simulink model "sensorfusion_diffdrive_VW"  (R2020b)
settings: Solver=ode1  StartTime=0.0  StopTime=100  FixedStep=0.01  RelTol=1e-3
settings Model: Creator=ONLY-GOD  LastModifiedBy=ONLY-GOD

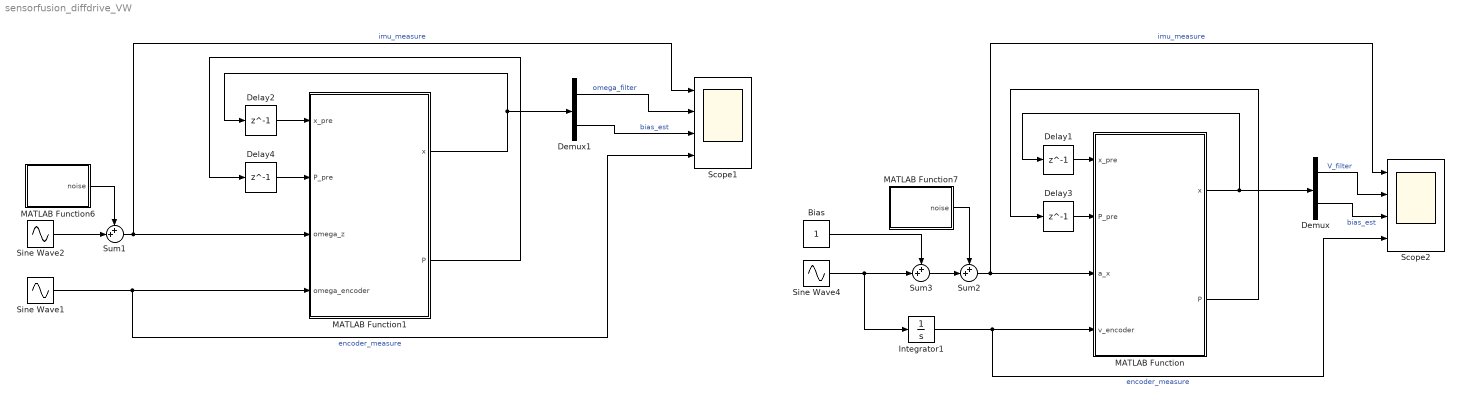
== system sensorfusion_diffdrive_VW ==
  Bias : Constant
  Delay1 : Delay  DelayLength=1  InitialCondition=[0;0]
  Delay2 : Delay  DelayLength=1  InitialCondition=[0;0]
  Delay3 : Delay  DelayLength=1  InitialCondition=2*eye(2);
  Delay4 : Delay  DelayLength=1  InitialCondition=2*eye(2);
  Demux : Demux  Outputs=2
  Demux1 : Demux  Outputs=2
  Integrator1 : Integrator
  MATLAB Function : MATLAB Function  TreatAsAtomicUnit=on
  MATLAB Function1 : MATLAB Function  TreatAsAtomicUnit=on
  MATLAB Function6 : MATLAB Function  TreatAsAtomicUnit=on
  MATLAB Function7 : MATLAB Function  TreatAsAtomicUnit=on
  Scope1 : Scope  NumInputPorts=4
  Scope2 : Scope  NumInputPorts=4
  Sine Wave1 : Sin  Amplitude=5  Frequency=0.1
  Sine Wave2 : Sin  Amplitude=5  Bias=1  Frequency=0.1
  Sine Wave4 : Sin  Amplitude=5  Frequency=0.1
  Sum1 : Sum  Inputs=++|
  Sum2 : Sum  Inputs=++|
  Sum3 : Sum  Inputs=++|
  wires:
  MATLAB Function/1(x) -> Delay1/1, Demux/1
  Demux/1 -> Scope2/2  "V_filter"
  Demux/2 -> Scope2/3  "bias_est"
  MATLAB Function/2(P) -> Delay3/1
  Delay3/1 -> MATLAB Function/2(P_pre)
  Delay1/1 -> MATLAB Function/1(x_pre)
  Delay2/1 -> MATLAB Function1/1(x_pre)
  MATLAB Function1/2(P) -> Delay4/1
  MATLAB Function1/1(x) -> Demux1/1, Delay2/1
  Delay4/1 -> MATLAB Function1/2(P_pre)
  Demux1/2 -> Scope1/3  "bias_est"
  Sine Wave1/1 -> Scope1/4, MATLAB Function1/4(omega_encoder)  "encoder_measure"
  Sum1/1 -> Scope1/1, MATLAB Function1/3(omega_z)  "imu_measure"
  Demux1/1 -> Scope1/2  "omega_filter"
  Sum2/1 -> Scope2/1, MATLAB Function/3(a_x)  "imu_measure"
  Integrator1/1 -> Scope2/4, MATLAB Function/4(v_encoder)  "encoder_measure"
  MATLAB Function7/1(noise) -> Sum2/1
  Sum3/1 -> Sum2/2
  Sine Wave4/1 -> Sum3/2, Integrator1/1
  Bias/1 -> Sum3/1
  Sine Wave2/1 -> Sum1/2
  MATLAB Function6/1(noise) -> Sum1/1

== matlab function sensorfusion_diffdrive_VW/MATLAB Function ==
  data: x_pre input; P_pre input; a_x input; x output; v_encoder input; P output
function [x,P] = kalman_V(x_pre,P_pre,a_x,v_encoder)
% predefined
Ts = 0.01;
Q = 1e-1*diag([2 2]);
R = 1e-3;
% model prediction
A = [1 Ts;
     0 1];
B = [Ts;
     0];
C = [1 0];

u = a_x;

x = A*x_pre + B*u;   %(2x1) = (2x2)(2x1) + (2x1)(1x1) checked
P = A*P_pre*A' + Q;  %(2x2) = (2x2)(2x2)(2x2) + (2x2) checked

%update
erry = v_encoder - C*x;      %(1x1) = (1x1) + (1x2)(2x1) checked
P_xz = P*C';
P_zz = C*P*C' + R;
x = x + (P_xz/P_zz)*erry;
P = P - (P_xz/P_zz)*P_xz';

== matlab function sensorfusion_diffdrive_VW/MATLAB Function1 ==
  data: x_pre input; P_pre input; omega_z input; x output; omega_encoder input; P output
function [x,P] = kalman_omega(x_pre,P_pre,omega_z,omega_encoder)
% predefined
Ts = 0.01;
Q = 1e-1*diag([2 200]);
R = 1e-4;
% model prediction
A = [0 1;
     0 1];
B = [1;
     0];
C = [1 0];

u = omega_z;

x = A*x_pre + B*u;   %(2x1) = (2x2)(2x1) + (2x1)(1x1) checked
P = A*P_pre*A' + Q;  %(2x2) = (2x2)(2x2)(2x2) + (2x2) checked

%update
erry = omega_encoder - C*x;      %(1x1) = (1x1) + (1x2)(2x1) checked
P_xz = P*C';
P_zz = C*P*C' + R;
x = x + (P_xz/P_zz)*erry;
P = P - (P_xz/P_zz)*P_xz';

== matlab function sensorfusion_diffdrive_VW/MATLAB Function6 ==
  data: noise output
function noise = fnc()

noise = randn*0.1;

== matlab function sensorfusion_diffdrive_VW/MATLAB Function7 ==
  data: noise output
function noise = fnc()

noise = randn*0.1;
